simulink library "gyroscope_sim_lib"  (R2018b)
settings: Solver=VariableStepAuto  StartTime=0.0  StopTime=10.0  RelTol=1e-3
undefined symbols (not defined in the file): DiscIntNeverNeededParam
settings Model: Creator=colem  LastModifiedBy=colem

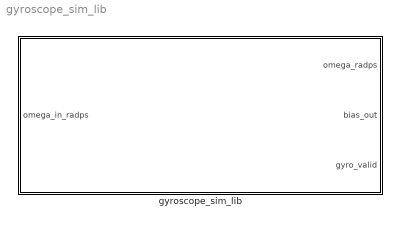
== system gyroscope_sim_lib ==
  gyroscope_sim_lib : Subsystem

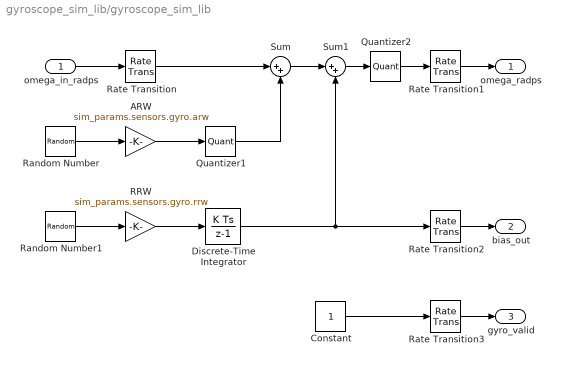
== system gyroscope_sim_lib/gyroscope_sim_lib ==
  omega_in_radps : Inport
  ARW : Gain  Gain=sim_params.sensors.gyro.arw
  Constant : Constant  SampleTime=sim_params.sensors.gyro.sample_time_s
  Discrete-Time Integrator : DiscreteIntegrator  InitialCondition=sim_params.sensors.gyro.bias_init  SampleTime=-1  ICPrevOutput=DiscIntNeverNeededParam  ICPrevScaledInput=DiscIntNeverNeededParam
  Quantizer1 : Quantizer  QuantizationInterval=sim_params.sensors.gyro.resolution
  Quantizer2 : Quantizer  QuantizationInterval=sim_params.sensors.gyro.resolution
  RRW : Gain  Gain=sim_params.sensors.gyro.rrw
  Random Number : RandomNumber  Mean=[0 0 0]  Variance=[1 1 1]  Seed=[77 88 99]  SampleTime=sim_params.sensors.gyro.sample_time_s
  Random Number1 : RandomNumber  Mean=[0 0 0]  Variance=[1 1 1]  Seed=[81 82 83]  SampleTime=sim_params.sensors.gyro.sample_time_s
  Rate Transition : RateTransition  InitialCondition=sim_params.dynamics.ic.rate_init  OutPortSampleTime=sim_params.sensors.gyro.sample_time_s
  Rate Transition1 : RateTransition  InitialCondition=sim_params.dynamics.ic.rate_init
  Rate Transition2 : RateTransition  InitialCondition=sim_params.sensors.gyro.bias_init
  Rate Transition3 : RateTransition  InitialCondition=1
  Sum : Sum  Inputs=|++
  Sum1 : Sum  Inputs=|++
  omega_radps : Outport
  bias_out : Outport  Port=2
  gyro_valid : Outport  Port=3
  wires:
  Random Number/1 -> ARW/1
  Random Number1/1 -> RRW/1
  ARW/1 -> Quantizer1/1
  omega_in_radps/1 -> Rate Transition/1
  Sum/1 -> Sum1/1
  RRW/1 -> Discrete-Time Integrator/1
  Constant/1 -> Rate Transition3/1
  Discrete-Time Integrator/1 -> Rate Transition2/1, Sum1/2
  Quantizer1/1 -> Sum/2
  Sum1/1 -> Quantizer2/1
  Quantizer2/1 -> Rate Transition1/1
  Rate Transition/1 -> Sum/1
  Rate Transition1/1 -> omega_radps/1
  Rate Transition2/1 -> bias_out/1
  Rate Transition3/1 -> gyro_valid/1
